simulink model "buck_pv"  (R2024a)
settings: Solver=FixedStepDiscrete  StartTime=0  StopTime=0.2  FixedStep=(1/150000)/100  RelTol=1e-3
model workspace (MAT data in the model file):
  Var = 20
libraries: spsSeriesRLCBranchLib x3, spsDiodeLib x2, spsMeanLib x2, spsCurrentMeasurementLib x1, spsDCVoltageSourceLib x1, spsGroundLib x1, spsMosfetLib x1, spsPVArrayLib x1, spsPWMGeneratorDCDCLib x1, spsVoltageMeasurementLib x1, spspowerguiLib x1
settings Model: Creator=mario  LastModifiedBy=mario
settings SolverCC: MaxConsecutiveMinStep=10  ZeroCrossAlgorithm=Adaptive  SolverResetMethod=Robust
settings DebuggingCC: IgnoredZcDiagnostic=none
settings ModelReferenceCC: EnableRefExpFcnMdlSchedulingChecks=on
settings RTWCC: GPUComputeCapability=3.5

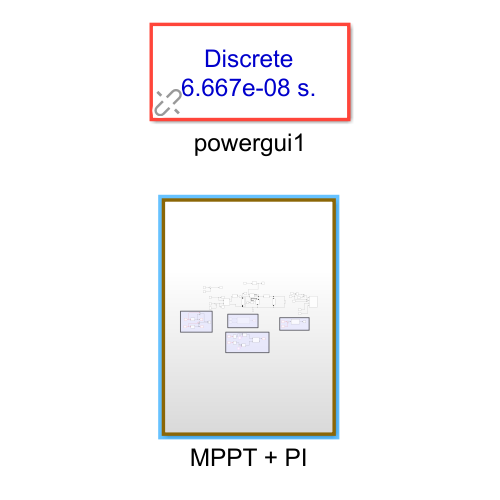
[thumbnail: Simulink's stored preview of the top-level diagram]
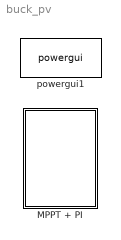
== system buck_pv ==
  MPPT + PI : Subsystem
  powergui1 : spspowerguiLib/powergui  Priority=1  SimulationMode=Discrete  SampleTime=(1/150000)/100  frequency=60  Iterations=50  frequencyindice=0  Pbase=100e6  ErrMax=1e-4  UnitsV=kV  UnitsW=MW  buscounter=0  FunctionMessages=off  echomessages=off  EnableUseOfTLC=off  CurrentSourceSwitches=off  DisableSnubberDevices=on  DisableRonSwitches=off  DisableVfSwitches=off  DisplayEquations=off  AutomaticDiscreteSolvers=off  SolverType=Tustin/Backward Euler (TBE)  Interpol=off  ExternalGateDelay=off  methode=off  Ts=100  x0status=blocks  SPID=on  SwTol=0  HookPort=off  NonlinearTolerance=1e-4  nMaxIteration=100  ContinueOnMaxIteration=on  RestoreLinks=warning  ResistiveCurrentMeasurement=off  Frange=[0:2:500]  Ylog=off  Xlog=on  ShowGrid=off  save=off  variable=ZData  structure=0  ZoomFFT=off  StartTime=0.0  cycles=1  DisplayStyle=1  fundamental=60  FreqAxis=off  MaxFrequency=1000  frequencyindicesteady=1  RmsSteady=1  display=off

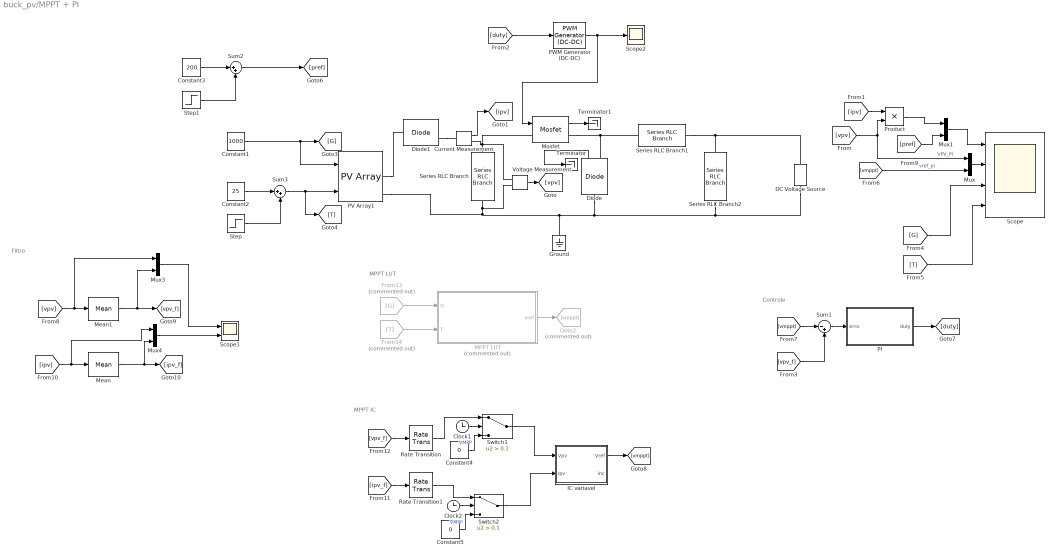
== system buck_pv/MPPT + PI ==
  note: MPPT IC
  note: MPPT LUT
  note: Filtro
  note: Controle
  Clock1 : Clock
  Clock2 : Clock
  Constant1 : Constant  Value=1000
  Constant2 : Constant  Value=25
  Constant3 : Constant  Value=200
  Constant4 : Constant  Value=0
  Constant5 : Constant  Value=0
  Current Measurement : spsCurrentMeasurementLib/Current Measurement  PhasorSimulation=off  OutputType=Complex  PSBequivalent=0
  DC Voltage Source : spsDCVoltageSourceLib/DC Voltage Source  Amplitude=12  Measurements=None
  Diode : spsDiodeLib/Diode  Ron=0.001  Lon=0  Vf=1  IC=0  UseSnubber=0  Rs=500  Cs=250e-9  Measurements=on
  Diode1 : spsDiodeLib/Diode  Ron=0.001  Lon=0  Vf=0.001  IC=0  UseSnubber=0  Rs=500  Cs=250e-9  Measurements=on
  From13 : From  Commented=on  GotoTag=G
  From14 : From  Commented=on  GotoTag=T
  Goto2 : Goto  Commented=on  GotoTag=vmppt
  Ground : spsGroundLib/Ground  LConnTagsString=a
  IC variavel : MATLAB Function  TreatAsAtomicUnit=on
  MPPT LUT : MATLAB Function  Commented=on  TreatAsAtomicUnit=on
  Mean : spsMeanLib/Mean  Freq=150e3  Vinit=0  Ts=1/150000/100
  Mean1 : spsMeanLib/Mean  Freq=150e3  Vinit=0  Ts=1/150000/100
  Mosfet : spsMosfetLib/Mosfet  Ron=0.15  Lon=0  Rd=0.01  Vfd=0  IC=0  Rs=1e5  Cs=inf  Measurements=on
  Mux{,1,3..4} (4 alike) : Mux  Inputs=2
  PI : Subsystem
  PV Array1 : spsPVArrayLib/PV Array  Npar=1  Nser=1  PlotType=array @ 25 deg.C & specified irradiances  S_vec="[ 1000  800 600 400 200]"  Temp_C_vec=[ 50 40 30 20 10 ]  ModuleName=User-defined  PlotWhenSelected=off  Pm=200.143  Ncell=45  Voc=32.9  Isc=8.21  Vm=26.3  Im=7.61  beta_Voc_pc=-0.32  alpha_Isc_pc=0.03177  beta_Voc=-0.10528  alpha_Isc=0.0026083  IL=8.311  I0=6.1007e-11  nI=1.112  Rsh=88.1591  Rs=0.36299  RobustModel=off  RobustCellTemperature=313.3991  BAL=off  Tc=1e-7  Tfilter=5e-5
  PWM Generator (DC-DC) : spsPWMGeneratorDCDCLib/PWM Generator (DC-DC)  Fsw=150000  Ts=1/150000/100
  Product : Product
  Rate Transition : RateTransition  OutPortSampleTime=30e-3
  Rate Transition1 : RateTransition  OutPortSampleTime=30e-3
  Scope : Scope  NumInputPorts=4
  Scope1 : Scope  NumInputPorts=2
  Scope2 : Scope
  Series RLC Branch : spsSeriesRLCBranchLib/Series RLC Branch  LConnTagsString=__new0  RConnTagsString=__new0  BranchType=RC  Resistance=6.519e-3  Inductance=1e-3  SetiL0=off  InitialCurrent=0  Capacitance=2.7e-3  Setx0=off  InitialVoltage=37.3  Measurements=None
  Series RLC Branch1 : spsSeriesRLCBranchLib/Series RLC Branch  LConnTagsString=__new0  RConnTagsString=__new0  BranchType=RL  Resistance=3e-3  Inductance=22.109e-6  SetiL0=off  InitialCurrent=25.8056  Capacitance=1e-6  Setx0=off  InitialVoltage=0  Measurements=None
  Series RLC Branch2 : spsSeriesRLCBranchLib/Series RLC Branch  LConnTagsString=__new0  RConnTagsString=__new0  BranchType=RC  Resistance=35.2e-3  Inductance=1e-3  SetiL0=off  InitialCurrent=0  Capacitance=500e-6  Setx0=off  InitialVoltage=12  Measurements=None
  Step : Step  Time=0.1  After=-10  SampleTime=0
  Step1 : Step  Time=0.1  After=7  SampleTime=0
  Sum1 : Sum  Inputs=|-+
  Sum2 : Sum  Inputs=|++
  Sum3 : Sum  Inputs=|++
  Switch1 : Switch  Criteria=u2 > Threshold  Threshold=0.1  SaturateOnIntegerOverflow=off  InputSameDT=off
  Switch2 : Switch  Criteria=u2 > Threshold  Threshold=0.1  SaturateOnIntegerOverflow=off  InputSameDT=off
  Terminator : Terminator
  Terminator1 : Terminator
  Voltage Measurement : spsVoltageMeasurementLib/Voltage Measurement  PhasorSimulation=off  OutputType=Complex  PSBequivalent=0
  wires:
  Mux1/1 -> Scope/1
  [ipv] -> Product/1
  PWM Generator (DC-DC)/1 -> Mosfet/1, Scope2/1
  [vpv] -> Product/2, Mux/1  "VPV_PI"
  [duty] -> PWM Generator (DC-DC)/1
  Product/1 -> Mux1/1
  [pref] -> Mux1/2
  [G] -> Scope/3
  [vmppt] -> Mux/2  "vref_pi"
  [T] -> Scope/4
  Mux/1 -> Scope/2
  Diode/1 -> Terminator/1
  Mosfet/1 -> Terminator1/1
  Voltage Measurement/1 -> [vpv]
  Current Measurement/1 -> [ipv]
  Mux4/1 -> Scope1/2
  Mux3/1 -> Scope1/1
  Mean1/1 -> Mux3/2, [vpv_f]
  [ipv] -> Mean/1, Mux4/1
  [vpv] -> Mean1/1, Mux3/1
  Mean/1 -> Mux4/2, [ipv_f]
  [vpv_f] -> Sum1/2
  [vmppt] -> Sum1/1
  Rate Transition1/1 -> Switch2/1
  Constant4/1 -> Switch1/3  "VMPP"
  Clock2/1 -> Switch2/2
  Rate Transition/1 -> Switch1/1
  Clock1/1 -> Switch1/2
  Switch2/1 -> IC variavel/2(Ipv)
  IC variavel/1(Vref) -> [vmppt]
  Switch1/1 -> IC variavel/1(Vpv)
  Constant5/1 -> Switch2/3  "VMPP"
  [ipv_f] -> Rate Transition1/1
  [vpv_f] -> Rate Transition/1
  Sum3/1 -> PV Array1/2, [T]
  Constant2/1 -> Sum3/1
  Constant1/1 -> PV Array1/1, [G]
  Sum1/1 -> PI/1(erro)
  PI/1(duty) -> [duty]
  From13/1 -> MPPT LUT/1(G)
  From14/1 -> MPPT LUT/2(T)
  MPPT LUT/1(vref) -> Goto2/1
  Step/1 -> Sum3/2
  Step1/1 -> Sum2/2
  Constant3/1 -> Sum2/1
  Sum2/1 -> [pref]
  connections:
  Series RLC Branch1/RConn1 -- DC Voltage Source/RConn1 -- Series RLC Branch2/LConn1
  Mosfet/LConn1 -- Current Measurement/RConn1 -- Voltage Measurement/LConn1 -- Series RLC Branch/LConn1
  Ground/LConn1 -- DC Voltage Source/LConn1 -- Series RLC Branch2/RConn1 -- Diode/LConn1 -- PV Array1/RConn2 -- Voltage Measurement/LConn2 -- Series RLC Branch/RConn1
  Mosfet/RConn1 -- Series RLC Branch1/LConn1 -- Diode/RConn1
  Diode1/RConn1 -- Current Measurement/LConn1
  PV Array1/RConn1 -- Diode1/LConn1

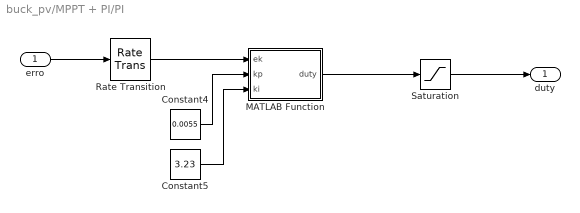
== system buck_pv/MPPT + PI/PI ==
  erro : Inport
  Constant4 : Constant  Value=0.0055
  Constant5 : Constant  Value=3.23
  MATLAB Function : MATLAB Function  TreatAsAtomicUnit=on
  Rate Transition : RateTransition  OutPortSampleTime=1/150000
  Saturation : Saturate  UpperLimit=1  LowerLimit=0
  duty : Outport
  wires:
  Saturation/1 -> duty/1
  Constant4/1 -> MATLAB Function/2(kp)
  Constant5/1 -> MATLAB Function/3(ki)
  MATLAB Function/1(duty) -> Saturation/1
  erro/1 -> Rate Transition/1
  Rate Transition/1 -> MATLAB Function/1(ek)

== matlab function buck_pv/MPPT + PI/PI/MATLAB Function ==
  settings: updateMethod=DISCRETE
  data: ek input; duty output; kp input; ki input
function duty = fcn(ek, kp, ki)

persistent uk_1 ek_1

if(isempty(uk_1)) uk_1=0; end
if(isempty(ek_1)) ek_1=0; end

Ts = (1/150e3);
A = kp + (ki*Ts/2);
B = kp - (ki*Ts/2);

u_PI = A*ek - B*ek_1 + uk_1;

ek_1 = ek;
uk_1 = u_PI;

duty = u_PI;

== matlab function buck_pv/MPPT + PI/IC variavel ==
  settings: sampleTime=30e-3
  data: Vpv input; Vref output; Ipv input; inc output
%MPPT Condutância Incremental com Passo Variável
function [Vref, inc]= f(Vpv, Ipv)
Vref_ini = 26.3; %tensão de referência inicial
k=0.1; %fator de incremento de vref

persistent Vpva Vrefa Ipva;

if isempty(Vpva) %testa se as variáveis ainda não foram inicializadas
 Vpva=0;
 Ipva=0;
 Vrefa=Vref_ini;
end

dV = Vpv - Vpva; %variação de tensão
dI = Ipv - Ipva; %variação de corrente
dP = (Vpv*Ipv - (Vpva*Ipva))/dV; %variação de potência

if isnan(dP) dP = 0; end
if (dP>20) dP = 0; end

% calculo do incremento variável
inc  = k*dP;

% saturação do incremento variável
if inc > 1
    inc = 1;
end
if inc < -1
    inc = -1;
end

Vref = Vrefa + inc;

if Vref > 35
    Vref = 35;
end
if Vref < 20
    Vref = 20;
end


Vpva=Vpv;
Ipva=Ipv;
Vrefa = Vref;
end

== matlab function buck_pv/MPPT + PI/MPPT LUT ==
  settings: updateMethod=DISCRETE  sampleTime=(1/150e3)
  data: G input; T input; vref output
function vref = fcn(G, T)

    persistent V_MPP V_MPP_aux P_MPP vpv;

    if(isempty(V_MPP)); V_MPP = 25; end
    if(isempty(V_MPP_aux)); V_MPP_aux = 0; end
    if(isempty(P_MPP)); P_MPP = 159.543; end
    if(isempty(vpv)); vpv = 0.1; end

    ipv = ipv_f(G, T, vpv);

    if(ipv<0); ipv = 0; end
    ppv = vpv*ipv

    if(ppv > P_MPP)
        V_MPP_aux = vpv;
        P_MPP = ppv;
    end
    if(vpv > 50)
        V_MPP = V_MPP_aux;
        P_MPP = 0;
        vpv = 0.1;
    end
    vref = V_MPP;
    vpv = vpv + 0.1;

end
